simulink model "Final_DellaVedova_RealimStateSpace2021"  (R2021a)
settings: Solver=VariableStepAuto  StartTime=0.0  StopTime=10.0  RelTol=1e-3
values from neighbouring files (symbols this model uses):
  K = Ka(1:order(G))    [final_problema_4.m]
  kI = -Ka(end)    [final_problema_4.m]
settings Model: Creator=aghersin  LastModifiedBy=maxirodriguez
settings SolverCC: AlgebraicLoopSolver=TrustRegion
settings DataIOCC: ReturnWorkspaceOutputs=off
settings DebuggingCC: ArithmeticOperatorsInVariantConditions=warning
settings SFSimCC: SimUseLocalCustomCode=off  CustomCodeUndefinedFunction=UseInterfaceOnly
settings RTWCC: RTWUseLocalCustomCode=off
settings CodeAppCC: StateflowObjectComments=on

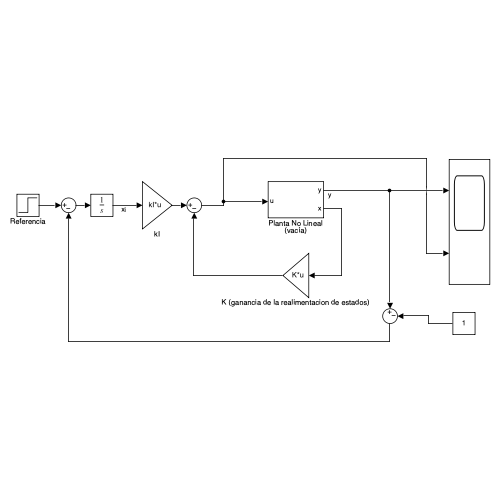
[thumbnail: Simulink's stored preview of the top-level diagram]
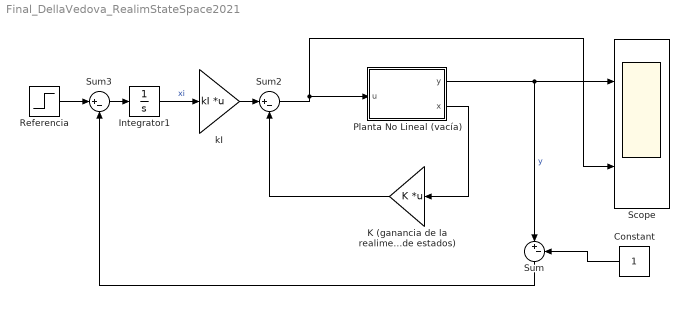
== system Final_DellaVedova_RealimStateSpace2021 ==
  Constant : Constant
  Integrator1 : Integrator
  K (ganancia de la realimentacion de estados) : Gain  Gain=K  Multiplication=Matrix(K*u)
  Planta No Lineal (vacía) : Subsystem
  Referencia : Step  After=0.1  SampleTime=0
  Scope : Scope  NumInputPorts=2
  Sum : Sum  Inputs=|+-
  Sum2 : Sum  Inputs=|+-
  Sum3 : Sum  Inputs=|+-
  kI : Gain  Gain=kI  Multiplication=Matrix(K*u)
  wires:
  Referencia/1 -> Sum3/1
  Sum2/1 -> Planta No Lineal (vacía)/1(u), Scope/2
  Sum3/1 -> Integrator1/1
  K (ganancia de la realimentacion de estados)/1 -> Sum2/2
  kI/1 -> Sum2/1
  Integrator1/1 -> kI/1  "xi"
  Planta No Lineal (vacía)/2(x) -> K (ganancia de la realimentacion de estados)/1
  Planta No Lineal (vacía)/1(y) -> Sum/1, Scope/1  "y"
  Sum/1 -> Sum3/2
  Constant/1 -> Sum/2

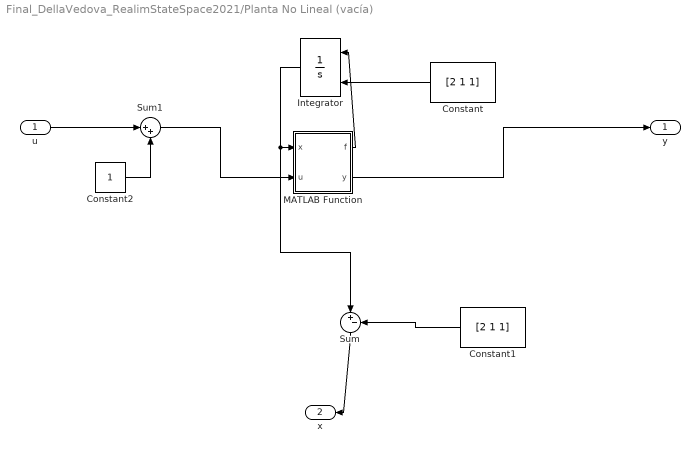
== system Final_DellaVedova_RealimStateSpace2021/Planta No Lineal (vacía) ==
  u : Inport
  Constant : Constant  Value=[2 1 1]
  Constant1 : Constant  Value=[2 1 1]
  Constant2 : Constant
  Integrator : Integrator  InitialConditionSource=external
  MATLAB Function : MATLAB Function  TreatAsAtomicUnit=on
  Sum : Sum  Inputs=|+-
  Sum1 : Sum  Inputs=|++
  y : Outport
  x : Outport  Port=2
  wires:
  MATLAB Function/1(f) -> Integrator/1
  Integrator/1 -> Sum/1, MATLAB Function/1(x)
  MATLAB Function/2(y) -> y/1
  Constant/1 -> Integrator/2
  Constant1/1 -> Sum/2
  Sum/1 -> x/1
  u/1 -> Sum1/1
  Sum1/1 -> MATLAB Function/2(u)
  Constant2/1 -> Sum1/2

== matlab function Final_DellaVedova_RealimStateSpace2021/Planta No Lineal (vacía)/MATLAB Function ==
  data: x input; f output; y output; u input
function [f,y] = fcn(x, u)

f1=(x(3) - sqrt(x(1)-x(2)))/x(1)^2;
f2=(sqrt(x(1)-x(2)) - sqrt(x(2)))/x(2)^2;
f3=0.02*(u-x(3));

f=[f1;f2;f3];

y=x(2);
